simulink model "work_1"  (R2022b)
settings: Solver=VariableStepAuto  StartTime=0.0  StopTime=20  RelTol=1e-3
values from neighbouring files (symbols this model uses):
  A = [-1 0 0 0;2 -3 0 0;0 0 2 0;4 -1 2 -4]    [work_.m]
  B = [0;0;1;2]    [work_.m]
  C = [3 0 1 0]    [work_.m]
  G = K4'    [work_.m]
settings Model: Creator=lifenghe  LastModifiedBy=acer
settings SolverCC: AlgebraicLoopSolver=TrustRegion
settings DataIOCC: ReturnWorkspaceOutputs=off
settings DebuggingCC: UnconnectedInputMsg=warning  UnconnectedOutputMsg=warning  UnconnectedLineMsg=warning  SFMachineParentedDataDiag=warning  ArithmeticOperatorsInVariantConditions=warning
settings ModelReferenceCC: EnableRefExpFcnMdlSchedulingChecks=on
settings SFSimCC: SimUseLocalCustomCode=off  CustomCodeUndefinedFunction=UseInterfaceOnly
settings RTWCC: RTWUseLocalCustomCode=off
settings CodeAppCC: StateflowObjectComments=on

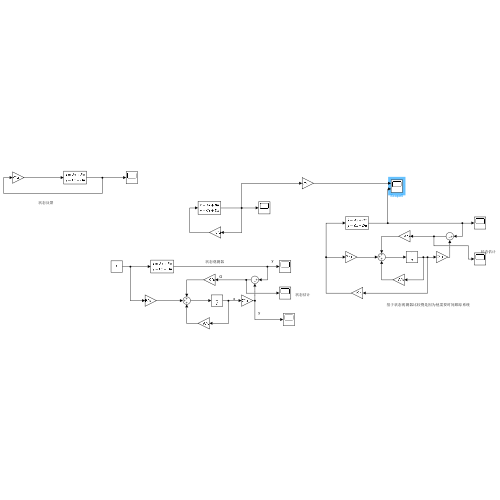
[thumbnail: Simulink's stored preview of the top-level diagram]
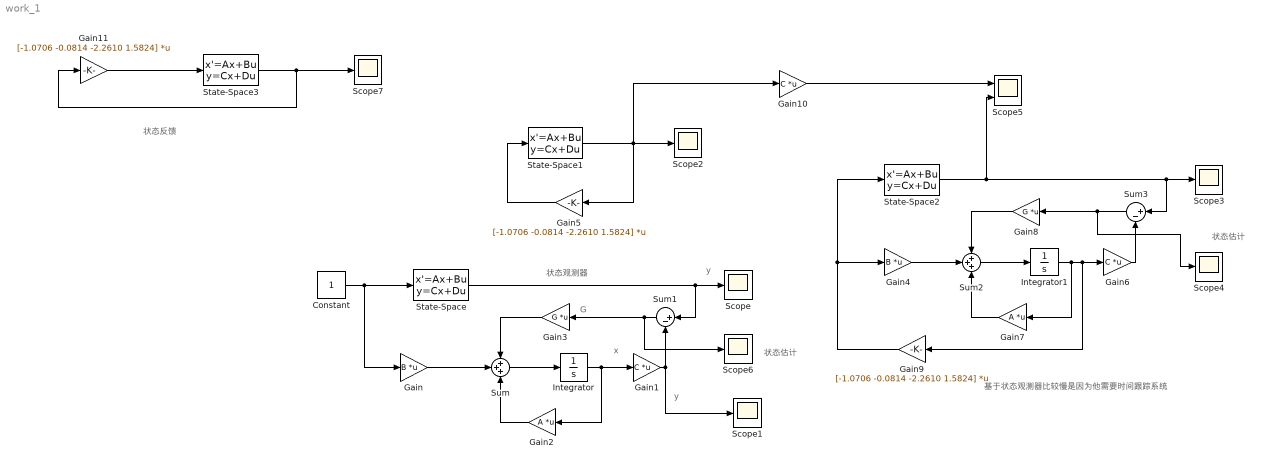
== system work_1 ==
  note: 状态反馈
  note: 基于状态观测器比较慢是因为他需要时间跟踪系统
  note: 状态估计
  note: y
  note: G
  note: x
  note: y
  note: 状态观测器
  note: 状态估计
  Constant : Constant
  Gain : Gain  Gain=B  Multiplication=Matrix(K*u)
  Gain1 : Gain  Gain=C  Multiplication=Matrix(K*u)
  Gain10 : Gain  Gain=C  Multiplication=Matrix(K*u)
  Gain11 : Gain  Gain=[-1.0706 -0.0814 -2.2610 1.5824]  Multiplication=Matrix(K*u)
  Gain2 : Gain  Gain=A  Multiplication=Matrix(K*u)
  Gain3 : Gain  Gain=G  Multiplication=Matrix(K*u)
  Gain4 : Gain  Gain=B  Multiplication=Matrix(K*u)
  Gain5 : Gain  Gain=[-1.0706 -0.0814 -2.2610 1.5824]  Multiplication=Matrix(K*u)
  Gain6 : Gain  Gain=C  Multiplication=Matrix(K*u)
  Gain7 : Gain  Gain=A  Multiplication=Matrix(K*u)
  Gain8 : Gain  Gain=G  Multiplication=Matrix(K*u)
  Gain9 : Gain  Gain=[-1.0706 -0.0814 -2.2610 1.5824]  Multiplication=Matrix(K*u)
  Integrator : Integrator
  Integrator1 : Integrator
  Scope{,1..4,6..7} (7 alike) : Scope
  Scope5 : Scope  NumInputPorts=2
  State-Space : StateSpace  A=[-1 0 0 0;2 -3 0 0;0 0 2 0;4 -1 2 -4]  B=[0;0;1;2]  C=C  D=0  InitialCondition=[0.1 0.2 0.3 0.4]
  State-Space1 : StateSpace  A=[-1 0 0 0;2 -3 0 0;0 0 2 0;4 -1 2 -4]  B=[0;0;1;2]  C=[1 0 0 0;0 1 0 0;0 0 1 0;0 0 0 1]  D=[0;0;0;0]  InitialCondition=[0.1 0.2 0.3 0.4]
  State-Space2 : StateSpace  A=[-1 0 0 0;2 -3 0 0;0 0 2 0;4 -1 2 -4]  B=[0;0;1;2]  C=C  D=0  InitialCondition=[0.1 0.2 0.3 0.4]
  State-Space3 : StateSpace  A=[-1 0 0 0;2 -3 0 0;0 0 2 0;4 -1 2 -4]  B=[0;0;1;2]  C=[1 0 0 0;0 1 0 0;0 0 1 0;0 0 0 1]  D=[0;0;0;0]  InitialCondition=[0.1 0.2 0.3 0.4]
  Sum : Sum  Inputs=+++
  Sum1 : Sum  Inputs=|+-
  Sum2 : Sum  Inputs=+++
  Sum3 : Sum  Inputs=|+-
  wires:
  State-Space/1 -> Sum1/1, Scope/1
  Constant/1 -> Gain/1, State-Space/1
  Sum/1 -> Integrator/1
  Integrator/1 -> Gain2/1, Gain1/1
  Gain2/1 -> Sum/3
  Gain/1 -> Sum/2
  Sum1/1 -> Gain3/1, Scope6/1
  Gain3/1 -> Sum/1
  Gain1/1 -> Scope1/1, Sum1/2
  State-Space1/1 -> Gain10/1, Gain5/1, Scope2/1
  Gain5/1 -> State-Space1/1
  Gain8/1 -> Sum2/1
  Sum2/1 -> Integrator1/1
  Sum3/1 -> Scope4/1, Gain8/1
  Gain4/1 -> Sum2/2
  Gain6/1 -> Sum3/2
  State-Space2/1 -> Scope5/2, Sum3/1, Scope3/1
  Gain7/1 -> Sum2/3
  Integrator1/1 -> Gain7/1, Gain9/1, Gain6/1
  Gain9/1 -> Gain4/1, State-Space2/1
  Gain10/1 -> Scope5/1
  Gain11/1 -> State-Space3/1
  State-Space3/1 -> Gain11/1, Scope7/1
